simulink model "Proposed"  (R2024b)
settings: Solver=VariableStepAuto  StartTime=0.0  StopTime=1  RelTol=1e-3
undefined symbols (not defined in the file or in its folder): DiscIntNeverNeededParam, Ki, Kp, Ts
libraries: spsDiodeLib x6, spsIGBTDiodeLib x6, spsSeriesRLCBranchLib x5, powerlib_extras x3, spsThreePhaseVIMeasurementLib x3, spsSaturableTransformerLib x3, spsThreePhaseSeriesRLCBranchLib x2, spsMultimeterLib x1, spsThreePhaseProgrammableVoltageSourceLib x1, spsGroundLib x1, dspfdesign x1, spsUniversalBridgeLib x1
settings Model: VariantFading=off  Creator=skill  LastModifiedBy=skill
settings DebuggingCC: AlgebraicLoopMsg=none

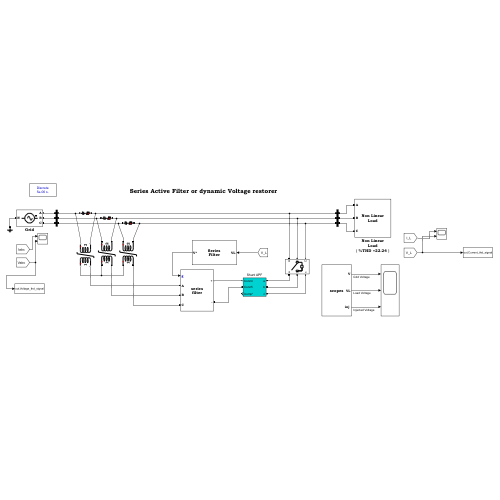
[thumbnail: Simulink's stored preview of the top-level diagram]
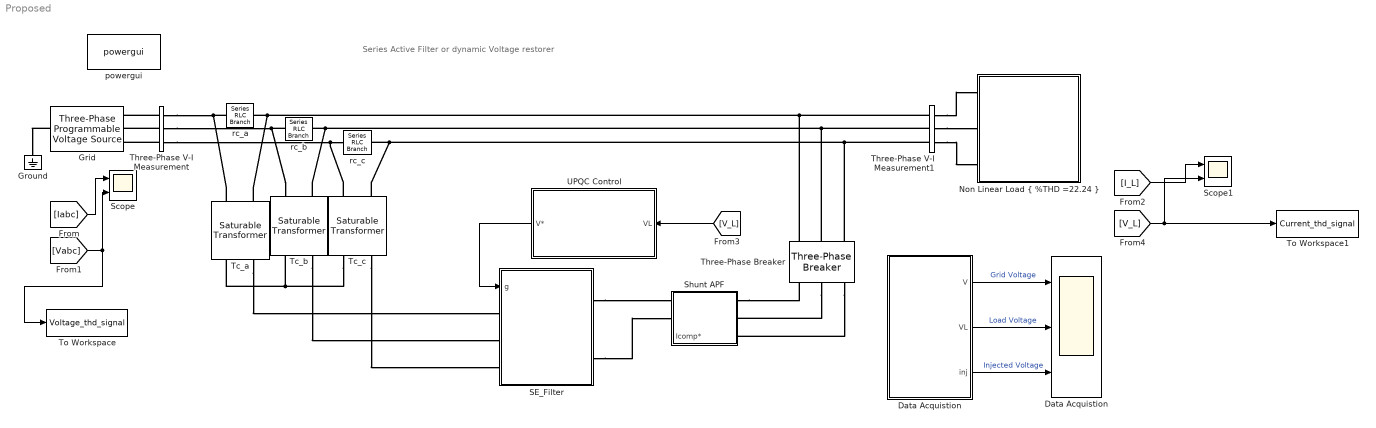
== system Proposed ==
  note: Series Active Filter or dynamic Voltage restorer
  Data Acquistion : Scope  NumInputPorts=3
  Data Acquistion : Subsystem
      mask Display: fprintf('scopes')
  Grid : spsThreePhaseProgrammableVoltageSourceLib/Three-Phase Programmable Voltage Source  PositiveSequence="[380  0 50]"  VariationEntity=Amplitude  VariationType=Table of time-amplitude pairs  VariationTypeAlt=Step  VariationStep=0.5  VariationRate=10  VariationMagnitude=0.3  VariationFrequency=2  VariationTiming=[1 2]  VariationPhaseA=off  Amplitudes=[1 0.5 1 1.5 1]  TimeValues=[0 0.5 0.7 1.5 1.7]  HarmonicGeneration=on  HarmonicA=[5 0.2 0 2]  HarmonicB=[7 0.05 0 1]  Timing="[0.2  0.4]"  BusType=swing  Pref=0  Qref=0  Qmin=-inf  Qmax=inf
  Ground : spsGroundLib/Ground  LConnTagsString=a
  "Non Linear Load { %THD =22.24 }" : Subsystem
      mask Display: fprintf('Non Linear\nLoad')
  SE_Filter : Subsystem
      mask Display: fprintf('series\nfilter')
  Scope : Scope  NumInputPorts=2
  Scope1 : Scope  NumInputPorts=2
  Shunt APF : Subsystem
      settings: PortSchema="{\"entries\":[{\"content\":{\"sides\":[{\"content\":{\"connectorIds\":[\"LConn1\",\"LConn2\",\"LConn3\"]},\"type\":\"ConnectorPlacement.EquallySpacedRectSide\",\"uuid\":\"d6bbf745-3af2-48b6-83a9-f1a4b39ae2fb\"},{\"content\":{\"connectorIds\":[\"RConn1\",\"RConn2\",\"Out1\"],\"side\":\"RIGHT\"},\"type\":\"ConnectorPlacement.EquallySpacedRectSide\",\"uuid\":\"e94a56cb-32a6-4b87-b27c-70bac7a36721\"},{\"content\":{\"side\":\"TOP\"},\"type\":\"ConnectorPlacement.EquallySpacedRectSide\",\"uuid\":\"720601aa-3b64-4420-8a99-8d6df25a17e3\"}]},\"type\":\"ConnectorPlacement.EquallySpacedConnector\",\"uuid\":\"c84ba404-e5ea-4b21-b879-47ad5a70dfc8\"}],\"packageUris\":[\"http://schema.mathworks.com/mf0/Connector/R2020b\"],\"version\":\"1.0\"}"
  Tc_a : spsSaturableTransformerLib/Saturable Transformer  ThreeWindings=off  Hysteresis=off  DataFile='hysteresis.mat'  Measurements=None  UNITS=pu  NominalPower=[4000 50]  Winding1="[380  0.02  0.02 ]"  Winding2="[380  0.02  0.02]"  Winding3="[ 315e3  0.002  0.08 ]"  Saturation=[ 0 0 ;1.016 9.043]*1e-3  CoreLoss=[117 0]  BreakLoop=off  DiscreteSolver=Trapezoidal iterative  DataType=off  InitialFlux=0  TransfoNumber=1
      settings: LibrarySourceBlock=sps_lib/Power Grid Elements/Saturable Transformer
  Tc_b : spsSaturableTransformerLib/Saturable Transformer  ThreeWindings=off  Hysteresis=off  DataFile='hysteresis.mat'  Measurements=None  UNITS=pu  NominalPower=[4000 50]  Winding1="[380  0.02  0.02 ]"  Winding2="[380  0.02  0.02]"  Winding3="[ 315e3  0.002  0.08 ]"  Saturation=[ 0 0 ;1.016 9.043]*1e-3  CoreLoss=[117 0]  BreakLoop=off  DiscreteSolver=Trapezoidal iterative  DataType=off  InitialFlux=0  TransfoNumber=1
      settings: LibrarySourceBlock=sps_lib/Power Grid Elements/Saturable Transformer
  Tc_c : spsSaturableTransformerLib/Saturable Transformer  ThreeWindings=off  Hysteresis=off  DataFile='hysteresis.mat'  Measurements=None  UNITS=pu  NominalPower=[4000 50]  Winding1="[380  0.02  0.02 ]"  Winding2="[380  0.02  0.02]"  Winding3="[ 315e3  0.002  0.08 ]"  Saturation=[ 0 0 ;1.016 9.043]*1e-3  CoreLoss=[117 0]  BreakLoop=off  DiscreteSolver=Trapezoidal iterative  DataType=off  InitialFlux=0  TransfoNumber=1
      settings: LibrarySourceBlock=sps_lib/Power Grid Elements/Saturable Transformer
  Three-Phase V-I Measurement : spsThreePhaseVIMeasurementLib/Three-Phase V-I Measurement  VoltageMeasurement=phase-to-ground  SetLabelV=on  LabelV=Vabc  Vpu=off  VpuLL=off  CurrentMeasurement=yes  SetLabelI=on  LabelI=Iabc  Ipu=off  Pbase=100e6  Vbase=500e3  OutputType=Complex  PhasorSimulation=off  PSBequivalent=0
  Three-Phase V-I Measurement1 : spsThreePhaseVIMeasurementLib/Three-Phase V-I Measurement  VoltageMeasurement=phase-to-ground  SetLabelV=on  LabelV=V_L  Vpu=off  VpuLL=off  CurrentMeasurement=yes  SetLabelI=on  LabelI=I_L  Ipu=off  Pbase=100e6  Vbase=500e3  OutputType=Complex  PhasorSimulation=off  PSBequivalent=0
  Three-Phase Breaker : spsThreePhaseBreakerLib/Three-Phase Breaker  InitialState=open  SwitchA=on  SwitchB=on  SwitchC=on  SwitchTimes=0.02  External=off  BreakerResistance=1e-6  SnubberResistance=1e6  SnubberCapacitance=inf  Measurements=None
  To Workspace : ToWorkspace  VariableName=Voltage_thd_signal  SaveFormat=Timeseries  SampleTime=-1
  To Workspace1 : ToWorkspace  VariableName=Current_thd_signal  SaveFormat=Timeseries  SampleTime=-1
  UPQC Control : Subsystem
      mask Display: fprintf('Series\nFilter')
  powergui : sps_lib/powergui  Priority=1  SimulationMode=Discrete  SampleTime=5e-6  frequency=60  Iterations=50  frequencyindice=50  Pbase=100e6  ErrMax=1e-4  UnitsV=kV  UnitsW=MW  buscounter=0  FunctionMessages=off  echomessages=off  EnableUseOfTLC=off  CurrentSourceSwitches=off  DisableSnubberDevices=off  DisableRonSwitches=off  DisableVfSwitches=off  DisplayEquations=off  AutomaticDiscreteSolvers=off  SolverType=Tustin/Backward Euler (TBE)  Interpol=off  ExternalGateDelay=off  methode=off  Ts=100  x0status=blocks  SPID=on  SwTol=0  HookPort=off  NonlinearTolerance=1e-4  nMaxIteration=100  ContinueOnMaxIteration=off  RestoreLinks=warning  ResistiveCurrentMeasurement=off  Frange=[0:2:500]  Ylog=off  Xlog=on  ShowGrid=off  save=off  variable=ZData  structure=0  ZoomFFT=off  StartTime=0.0  cycles=1  DisplayStyle=1  fundamental=60  FreqAxis=off  MaxFrequency=1000  frequencyindicesteady=1  RmsSteady=1  display=off
  rc_a : spsSeriesRLCBranchLib/Series RLC Branch  LConnTagsString=__new0  RConnTagsString=__new0  BranchType=RC  Resistance=1  Inductance=1e-3  SetiL0=off  InitialCurrent=0  Capacitance=100e-6  Setx0=off  InitialVoltage=0  Measurements=Branch voltage
  rc_b : spsSeriesRLCBranchLib/Series RLC Branch  LConnTagsString=__new0  RConnTagsString=__new0  BranchType=RC  Resistance=1  Inductance=1e-3  SetiL0=off  InitialCurrent=0  Capacitance=100e-6  Setx0=off  InitialVoltage=0  Measurements=Branch voltage
  rc_c : spsSeriesRLCBranchLib/Series RLC Branch  LConnTagsString=__new0  RConnTagsString=__new0  BranchType=RC  Resistance=1  Inductance=1e-3  SetiL0=off  InitialCurrent=0  Capacitance=100e-6  Setx0=off  InitialVoltage=0  Measurements=Branch voltage
  wires:
  Data Acquistion/1(V) -> Data Acquistion/1  "Grid Voltage"
  Data Acquistion/2(VL) -> Data Acquistion/2  "Load Voltage"
  [V_L] -> UPQC Control/1(VL)
  UPQC Control/1(V*) -> SE_Filter/1(g)
  Data Acquistion/3("inj ") -> Data Acquistion/3  "Injected Voltage"
  [Iabc] -> Scope/1
  [Vabc] -> To Workspace/1, Scope/2
  [I_L] -> Scope1/1
  [V_L] -> Scope1/2, To Workspace1/1
  connections:
  Tc_c/RConn2 -- Three-Phase Breaker/LConn3 -- Three-Phase V-I Measurement1/LConn3 -- rc_c/LConn1
  Tc_a/RConn1 -- rc_a/RConn1 -- Three-Phase V-I Measurement/RConn1
  Tc_b/LConn1 -- Tc_c/LConn1 -- Tc_a/LConn1
  Tc_c/RConn1 -- rc_c/RConn1 -- Three-Phase V-I Measurement/RConn3
  Tc_a/RConn2 -- Three-Phase Breaker/LConn1 -- Three-Phase V-I Measurement1/LConn1 -- rc_a/LConn1
  Tc_b/RConn1 -- rc_b/RConn1 -- Three-Phase V-I Measurement/RConn2
  Tc_b/RConn2 -- Three-Phase Breaker/LConn2 -- Three-Phase V-I Measurement1/LConn2 -- rc_b/LConn1
  Three-Phase V-I Measurement1/RConn3 -- "Non Linear Load { %THD =22.24 }"/LConn3
  Three-Phase V-I Measurement/LConn1 -- Grid/RConn1
  Three-Phase V-I Measurement1/RConn1 -- "Non Linear Load { %THD =22.24 }"/LConn1
  Three-Phase V-I Measurement/LConn2 -- Grid/RConn2
  Tc_c/LConn2 -- SE_Filter/LConn3
  Tc_b/LConn2 -- SE_Filter/LConn2
  Three-Phase V-I Measurement/LConn3 -- Grid/RConn3
  Tc_a/LConn2 -- SE_Filter/LConn1
  Three-Phase V-I Measurement1/RConn2 -- "Non Linear Load { %THD =22.24 }"/LConn2
  Grid/LConn1 -- Ground/LConn1
  Three-Phase Breaker/RConn2 -- Shunt APF/LConn2
  Shunt APF/LConn1 -- Three-Phase Breaker/RConn1
  Three-Phase Breaker/RConn3 -- Shunt APF/LConn3
  SE_Filter/RConn1 -- Shunt APF/RConn1
  SE_Filter/RConn2 -- Shunt APF/RConn2

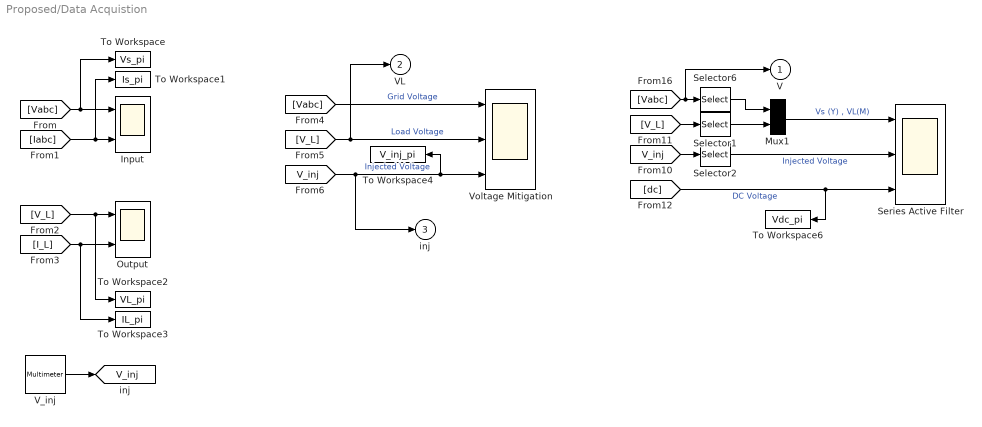
== system Proposed/Data Acquistion ==
  Input : Scope  NumInputPorts=2
  Mux1 : Mux  Inputs=2
      settings: DisplayOption=signals
  Output : Scope  NumInputPorts=2
  Selector1 : Selector  InputPortWidth=3  IndexOptions=Index vector (dialog)  Indices=1  OutputSizes=1
  Selector2 : Selector  InputPortWidth=3  IndexOptions=Index vector (dialog)  Indices=1  OutputSizes=1
  Selector6 : Selector  InputPortWidth=3  IndexOptions=Index vector (dialog)  Indices=1  OutputSizes=1
  Series Active Filter : Scope  NumInputPorts=3
  To Workspace : ToWorkspace  VariableName=Vs_pi  SampleTime=Ts
  To Workspace1 : ToWorkspace  VariableName=Is_pi  SampleTime=Ts
  To Workspace2 : ToWorkspace  VariableName=VL_pi  SampleTime=Ts
  To Workspace3 : ToWorkspace  VariableName=IL_pi  SampleTime=Ts
  To Workspace4 : ToWorkspace  VariableName=V_inj_pi  SampleTime=Ts
  To Workspace6 : ToWorkspace  VariableName=Vdc_pi  SampleTime=Ts
  V_inj : spsMultimeterLib/Multimeter  L=3  sel=[1 2 3]  yselected={}  Gain=[1 1 1]  OutputType=Complex  PlotAtSimulationStop=off  PhasorSimulation=off
  Voltage Mitigation : Scope  NumInputPorts=3
  V : Outport
  VL : Outport  Port=2
  "inj " : Outport  Port=3
  tag scope: V_inj=global
  wires:
  [Vabc] -> Input/1, To Workspace/1
  [Iabc] -> Input/2, To Workspace1/1
  [V_L] -> Output/1, To Workspace2/1
  [I_L] -> Output/2, To Workspace3/1
  [Vabc] -> Voltage Mitigation/1  "Grid Voltage"
  [V_L] -> Voltage Mitigation/2, VL/1  "Load Voltage"
  [V_inj] -> Voltage Mitigation/3, To Workspace4/1, "inj "/1  "Injected Voltage"
  [V_L] -> Selector1/1
  [V_inj] -> Selector2/1
  [dc] -> Series Active Filter/3, To Workspace6/1  "DC Voltage"
  Selector2/1 -> Series Active Filter/2  "Injected Voltage"
  [Vabc] -> Selector6/1, V/1
  Selector1/1 -> Mux1/2
  Mux1/1 -> Series Active Filter/1  "Vs (Y) , VL(M)"
  Selector6/1 -> Mux1/1
  V_inj/1 -> [V_inj]

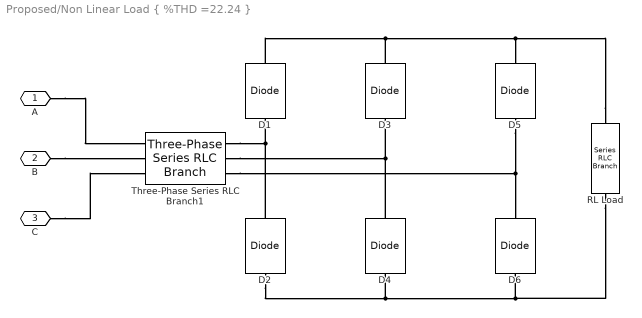
== system Proposed/Non Linear Load { %THD =22.24 } ==
  D{1..6} (6 alike) : spsDiodeLib/Diode  Ron=0.001  Lon=0  Vf=0.8  IC=0  UseSnubber=off  Rs=500  Cs=250e-9  Measurements=off
  RL Load : spsSeriesRLCBranchLib/Series RLC Branch  LConnTagsString=__new0  RConnTagsString=__new0  BranchType=RL  Resistance=60  Inductance=0.15e-3  SetiL0=off  InitialCurrent=0  Capacitance=1e-6  Setx0=off  InitialVoltage=0  Measurements=None
  Three-Phase Series RLC Branch1 : spsThreePhaseSeriesRLCBranchLib/Three-Phase Series RLC Branch  LConnTagsString=A|B|C  RConnTagsString=A|B|C  BranchType=RL  Resistance=0.4  Inductance=15e-3  Capacitance=1e-6  Measurements=None
  A : PMIOPort  Side=Left
  B : PMIOPort  Port=2  Side=Left
  C : PMIOPort  Port=3  Side=Left
  connections:
  C/RConn1 -- Three-Phase Series RLC Branch1/LConn3
  B/RConn1 -- Three-Phase Series RLC Branch1/LConn2
  A/RConn1 -- Three-Phase Series RLC Branch1/LConn1
  Three-Phase Series RLC Branch1/RConn3 -- D6/RConn1 -- D5/LConn1
  Three-Phase Series RLC Branch1/RConn2 -- D4/RConn1 -- D3/LConn1
  RL Load/RConn1 -- D6/LConn1 -- D4/LConn1 -- D2/LConn1
  RL Load/LConn1 -- D5/RConn1 -- D3/RConn1 -- D1/RConn1
  Three-Phase Series RLC Branch1/RConn1 -- D2/RConn1 -- D1/LConn1

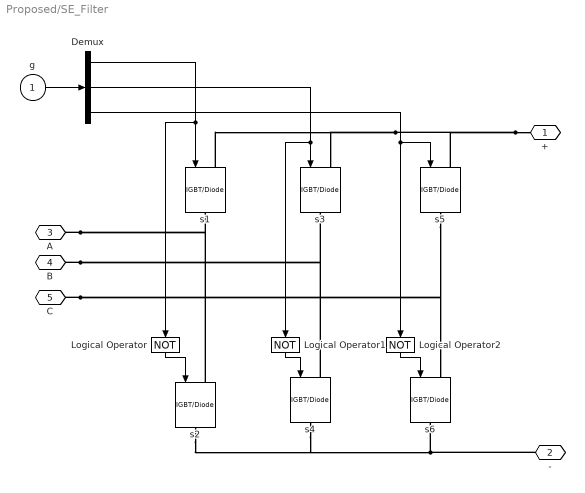
== system Proposed/SE_Filter ==
  g : Inport
  Demux : Demux  Outputs=3
      settings: DisplayOption=none
  Logical Operator : Logic  Operator=NOT  AllPortsSameDT=off  OutDataTypeStr=boolean
  Logical Operator1 : Logic  Operator=NOT  AllPortsSameDT=off  OutDataTypeStr=boolean
  Logical Operator2 : Logic  Operator=NOT  AllPortsSameDT=off  OutDataTypeStr=boolean
  s{1..6} (6 alike) : spsIGBTDiodeLib/IGBT//Diode  Ron=1e-3  Rs=1e5  Cs=inf  Measurements=off
  + : PMIOPort  Side=Right
  - : PMIOPort  Port=2  Side=Right
  A : PMIOPort  Port=3  Side=Left
  B : PMIOPort  Port=4  Side=Left
  C : PMIOPort  Port=5  Side=Left
  wires:
  Demux/2 -> s3/1, Logical Operator1/1
  Demux/1 -> s1/1, Logical Operator/1
  Logical Operator/1 -> s2/1
  Logical Operator1/1 -> s4/1
  Logical Operator2/1 -> s6/1
  Demux/3 -> Logical Operator2/1, s5/1
  g/1 -> Demux/1
  connections:
  +/RConn1 -- s5/LConn1 -- s1/LConn1 -- s3/LConn1
  A/RConn1 -- s2/LConn1 -- s1/RConn1
  -/RConn1 -- s6/RConn1 -- s4/RConn1 -- s2/RConn1
  B/RConn1 -- s4/LConn1 -- s3/RConn1
  C/RConn1 -- s5/RConn1 -- s6/LConn1

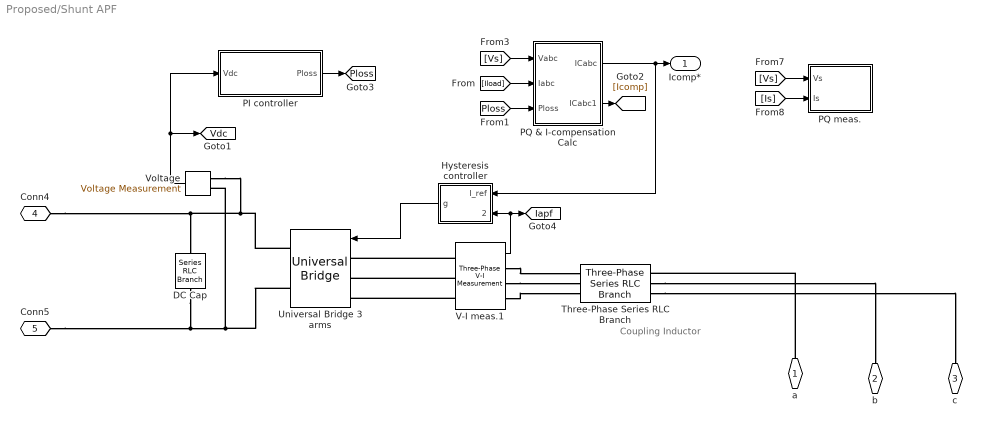
== system Proposed/Shunt APF ==
  note: Coupling Inductor
  DC Cap : spsSeriesRLCBranchLib/Series RLC Branch  LConnTagsString=__new0  RConnTagsString=__new0  BranchType=C  Resistance=1  Inductance=1e-3  SetiL0=off  InitialCurrent=0  Capacitance=3.5e-6  Setx0=off  InitialVoltage=400  Measurements=None
  Hysteresis controller : Subsystem
  PI controller : Subsystem
  PQ & I-compensation Calc : Subsystem
  PQ meas. : Subsystem
  Three-Phase Series RLC Branch : spsThreePhaseSeriesRLCBranchLib/Three-Phase Series RLC Branch  LConnTagsString=A|B|C  RConnTagsString=A|B|C  BranchType=L  Resistance=1e9  Inductance=10e-3  Capacitance=.2e-3  Measurements=None
  Universal Bridge 3 arms : spsUniversalBridgeLib/Universal Bridge  Arms=3  SnubberResistance=10000  SnubberCapacitance=inf  Device=IGBT / Diodes  Ron=1e-4  Lon=0  ForwardVoltages="[  1  1  ]"  ForwardVoltage=.8  GTOparameters=[ 10e-6 , 20e-6 ]  IGBTparameters=[ 1e-6 , 2e-6 ]  Measurements=None  Measurements_2=None  converterType=Rectifier
      settings: AttributesFormatString=\n
  V-I meas.1 : spsThreePhaseVIMeasurementLib/Three-Phase V-I Measurement  VoltageMeasurement=phase-to-ground  SetLabelV=on  LabelV=Vnm  Vpu=off  VpuLL=off  CurrentMeasurement=yes  SetLabelI=off  LabelI=Iabc  Ipu=off  Pbase=100e6  Vbase=500e3  OutputType=Complex  PhasorSimulation=off  PSBequivalent=0
  Voltage : spsVoltageMeasurementLib/Voltage Measurement  PhasorSimulation=off  OutputType=Complex  PSBequivalent=0
  a : PMIOPort  Side=Left
  b : PMIOPort  Port=2  Side=Left
  c : PMIOPort  Port=3  Side=Left
  Conn4 : PMIOPort  Port=4  Side=Right
  Conn5 : PMIOPort  Port=5  Side=Right
  Icomp* : Outport
  tag scope: Iapf=global, Ploss=global, Vdc=global
  wires:
  [Iload] -> PQ & I-compensation Calc/2(Iabc)
  V-I meas.1/1 -> Hysteresis controller/2(I_meas), [Iapf]
  Hysteresis controller/1(g) -> Universal Bridge 3 arms/1
  PQ & I-compensation Calc/1(ICabc) -> Hysteresis controller/1(I_ref), Icomp*/1
  Voltage/1 -> PI controller/1(Vdc), [Vdc]
  [Vs] -> PQ & I-compensation Calc/1(Vabc)
  PQ & I-compensation Calc/2(ICabc1) -> [Icomp]
  PI controller/1(Ploss) -> [Ploss]
  [Ploss] -> PQ & I-compensation Calc/3(Ploss)
  [Vs] -> PQ meas./1(Vs)
  [Is] -> PQ meas./2(Is)
  connections:
  Voltage/LConn1 -- DC Cap/LConn1 -- Conn4/RConn1 -- Universal Bridge 3 arms/RConn1
  V-I meas.1/LConn1 -- Universal Bridge 3 arms/LConn1
  V-I meas.1/LConn2 -- Universal Bridge 3 arms/LConn2
  V-I meas.1/RConn3 -- Three-Phase Series RLC Branch/LConn3
  V-I meas.1/RConn2 -- Three-Phase Series RLC Branch/LConn2
  V-I meas.1/LConn3 -- Universal Bridge 3 arms/LConn3
  V-I meas.1/RConn1 -- Three-Phase Series RLC Branch/LConn1
  a/RConn1 -- Three-Phase Series RLC Branch/RConn1
  Three-Phase Series RLC Branch/RConn2 -- b/RConn1
  Three-Phase Series RLC Branch/RConn3 -- c/RConn1
  DC Cap/RConn1 -- Conn5/RConn1 -- Universal Bridge 3 arms/RConn2 -- Voltage/LConn2

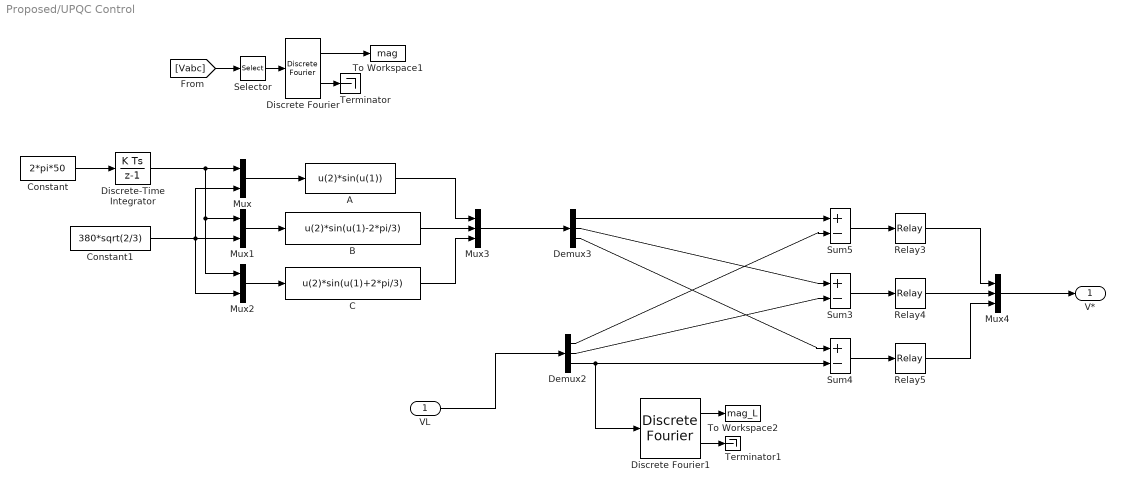
== system Proposed/UPQC Control ==
  VL : Inport
  A : Fcn  Expr=u(2)*sin(u(1))
  B : Fcn  Expr=u(2)*sin(u(1)-2*pi/3)
  C : Fcn  Expr=u(2)*sin(u(1)+2*pi/3)
  Constant : Constant  Value=2*pi*50
  Constant1 : Constant  Value=380*sqrt(2/3)
  Demux2 : Demux  Outputs=3
  Demux3 : Demux  Outputs=3
  Discrete Fourier : powerlib_extras/Discrete Measurements/Discrete  Fourier  Freq=50  n=1  Par_Init=[0 0]  Ts=Ts
  Discrete Fourier1 : powerlib_extras/Discrete Measurements/Discrete  Fourier  Freq=50  n=1  Par_Init=[0 0]  Ts=Ts
  Discrete-Time Integrator : DiscreteIntegrator  gainval=Gain  SampleTime=Ts  ICPrevOutput=DiscIntNeverNeededParam  ICPrevScaledInput=DiscIntNeverNeededParam
  Mux : Mux  Inputs=2
  Mux1 : Mux  Inputs=2
  Mux2 : Mux  Inputs=2
  Mux3 : Mux  Inputs=3
  Mux4 : Mux  Inputs=3
  Relay3 : Relay  OnSwitchValue=1  OffSwitchValue=-1
  Relay4 : Relay  OnSwitchValue=1  OffSwitchValue=-1
  Relay5 : Relay  OnSwitchValue=1  OffSwitchValue=-1
  Selector : Selector  InputPortWidth=3  IndexOptions=Index vector (dialog)  Indices=1  OutputSizes=1
  Sum3 : Sum  Inputs=+-
  Sum4 : Sum  Inputs=+-
  Sum5 : Sum  Inputs=+-
  Terminator : Terminator
  Terminator1 : Terminator
  To Workspace1 : ToWorkspace  VariableName=mag  SampleTime=Ts
  To Workspace2 : ToWorkspace  VariableName=mag_L  SampleTime=Ts
  V* : Outport
  wires:
  Constant/1 -> Discrete-Time Integrator/1
  Discrete-Time Integrator/1 -> Mux/1, Mux2/1, Mux1/1
  Constant1/1 -> Mux1/2, Mux2/2, Mux/2
  Mux/1 -> A/1
  Mux1/1 -> B/1
  Mux2/1 -> C/1
  Discrete Fourier/2 -> Terminator/1
  Selector/1 -> Discrete Fourier/1
  [Vabc] -> Selector/1
  Discrete Fourier/1 -> To Workspace1/1
  A/1 -> Mux3/1
  B/1 -> Mux3/2
  C/1 -> Mux3/3
  Discrete Fourier1/2 -> Terminator1/1
  Sum5/1 -> Relay3/1
  Sum3/1 -> Relay4/1
  Sum4/1 -> Relay5/1
  Relay3/1 -> Mux4/1
  Relay4/1 -> Mux4/2
  Relay5/1 -> Mux4/3
  Mux4/1 -> V*/1
  Discrete Fourier1/1 -> To Workspace2/1
  VL/1 -> Demux2/1
  Demux3/1 -> Sum5/1
  Demux2/3 -> Sum4/2, Discrete Fourier1/1
  Demux2/1 -> Sum5/2
  Demux3/3 -> Sum4/1
  Demux2/2 -> Sum3/2
  Demux3/2 -> Sum3/1
  Mux3/1 -> Demux3/1

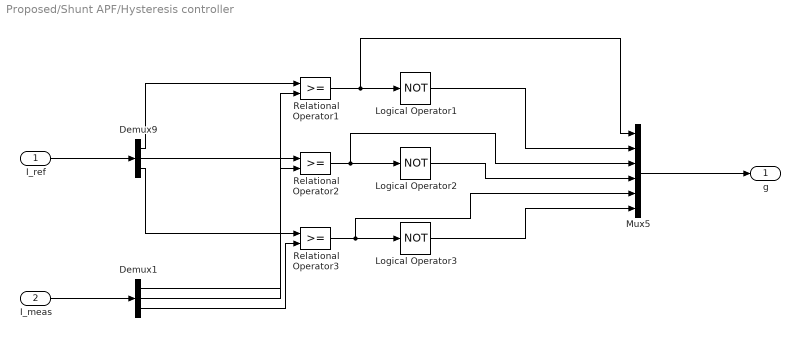
== system Proposed/Shunt APF/Hysteresis controller ==
  I_ref : Inport
  I_meas : Inport  Port=2
  Demux1 : Demux  Outputs=3
  Demux9 : Demux  Outputs=3
  Logical Operator1 : Logic  Operator=NOT  AllPortsSameDT=off  OutDataTypeStr=boolean
  Logical Operator2 : Logic  Operator=NOT  AllPortsSameDT=off  OutDataTypeStr=boolean
  Logical Operator3 : Logic  Operator=NOT  AllPortsSameDT=off  OutDataTypeStr=boolean
  Mux5 : Mux  Inputs=6
  Relational Operator1 : RelationalOperator  OutDataTypeStr=boolean  InputSameDT=off
  Relational Operator2 : RelationalOperator  OutDataTypeStr=boolean  InputSameDT=off
  Relational Operator3 : RelationalOperator  OutDataTypeStr=boolean  InputSameDT=off
  g : Outport
  wires:
  Relational Operator1/1 -> Logical Operator1/1, Mux5/1
  Relational Operator2/1 -> Logical Operator2/1, Mux5/3
  Relational Operator3/1 -> Logical Operator3/1, Mux5/5
  Demux9/1 -> Relational Operator1/1
  Demux9/3 -> Relational Operator3/1
  Logical Operator1/1 -> Mux5/2
  Logical Operator2/1 -> Mux5/4
  Logical Operator3/1 -> Mux5/6
  Mux5/1 -> g/1
  Demux9/2 -> Relational Operator2/1
  Demux1/1 -> Relational Operator1/2
  Demux1/2 -> Relational Operator2/2
  Demux1/3 -> Relational Operator3/2
  I_ref/1 -> Demux9/1
  I_meas/1 -> Demux1/1

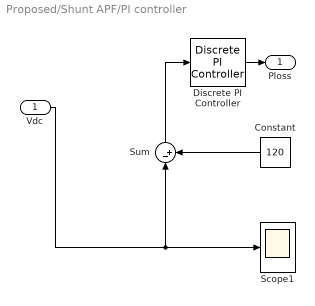
== system Proposed/Shunt APF/PI controller ==
  Vdc : Inport
  Constant : Constant  Value=120
  Discrete PI Controller : powerlib_extras/Discrete  Control Blocks/Discrete PI Controller  Kp=Kp  Ki=Ki  Par_Limits=[1e6 -1e6]  Init=0  Ts=5e-6
  Scope1 : Scope
  Sum : Sum  Inputs=|-+
  Ploss : Outport
  wires:
  Constant/1 -> Sum/2
  Sum/1 -> Discrete PI Controller/1
  Discrete PI Controller/1 -> Ploss/1
  Vdc/1 -> Sum/1, Scope1/1

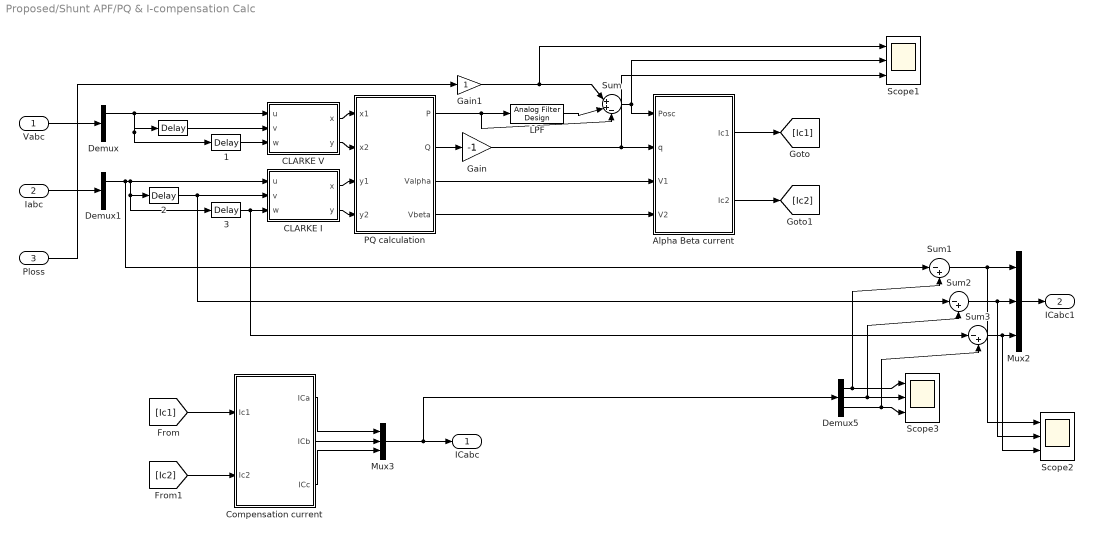
== system Proposed/Shunt APF/PQ & I-compensation Calc ==
  Vabc : Inport
  Iabc : Inport  Port=2
  Ploss : Inport  Port=3
  " " : TransportDelay  DelayTime=0.006666666  BufferSize=6890
  " 1" : TransportDelay  DelayTime=0.013333333  BufferSize=77889
  " 2" : TransportDelay  DelayTime=0.006666666  BufferSize=6789
  " 3" : TransportDelay  DelayTime=0.013333333  BufferSize=5667
  Alpha Beta current : MATLAB Function  TreatAsAtomicUnit=on
  CLARKE I : MATLAB Function  TreatAsAtomicUnit=on
  CLARKE V : MATLAB Function  TreatAsAtomicUnit=on
  Compensation current : MATLAB Function  TreatAsAtomicUnit=on
  Demux : Demux  Outputs=3
  Demux1 : Demux  Outputs=3
  Demux5 : Demux  Outputs=3
  Gain : Gain  Gain=-1
  Gain1 : Gain
  LPF : dspfdesign/Analog Filter Design  method=Butterworth  filttype=Lowpass  N=5  Wlo=2*pi*50  Whi=80  Rp=2  Rs=40
  Mux2 : Mux  Inputs=3
  Mux3 : Mux  Inputs=3
  PQ calculation : MATLAB Function  TreatAsAtomicUnit=on
  Scope1 : Scope  NumInputPorts=3
  Scope2 : Scope  NumInputPorts=3
  Scope3 : Scope  NumInputPorts=3
  Sum : Sum  Inputs=|++-
  Sum1 : Sum  Inputs=|-+
  Sum2 : Sum  Inputs=|-+
  Sum3 : Sum  Inputs=|-+
  ICabc : Outport
  ICabc1 : Outport  Port=2
  wires:
  Iabc/1 -> Demux1/1
  Vabc/1 -> Demux/1
  [Ic1] -> Compensation current/1(Ic1)
  [Ic2] -> Compensation current/2(Ic2)
  Compensation current/1(ICa) -> Mux3/1
  Compensation current/2(ICb) -> Mux3/2
  Compensation current/3(ICc) -> Mux3/3
  CLARKE V/1(x) -> PQ calculation/1(x1)
  CLARKE V/2(y) -> PQ calculation/2(x2)
  CLARKE I/1(x) -> PQ calculation/3(y1)
  PQ calculation/2(Q) -> Gain/1
  PQ calculation/1(P) -> LPF/1, Sum/3
  Gain/1 -> Alpha Beta current/2(q), Scope1/3
  PQ calculation/3(Valpha) -> Alpha Beta current/3(V1)
  Alpha Beta current/1(Ic1) -> [Ic1]
  Alpha Beta current/2(Ic2) -> [Ic2]
  CLARKE I/2(y) -> PQ calculation/4(y2)
  PQ calculation/4(Vbeta) -> Alpha Beta current/4(V2)
  Demux/1 -> CLARKE V/1(u), " "/1, " 1"/1
  Demux1/1 -> Sum1/1, CLARKE I/1(u), " 3"/1, " 2"/1
  LPF/1 -> Sum/2
  Sum/1 -> Alpha Beta current/1(Posc), Scope1/2
  Gain1/1 -> Sum/1, Scope1/1
  Mux3/1 -> ICabc/1, Demux5/1
  Demux5/1 -> Scope3/1, Sum1/2
  Demux5/2 -> Scope3/2, Sum2/2
  Demux5/3 -> Scope3/3, Sum3/2
  Ploss/1 -> Gain1/1
  Sum1/1 -> Mux2/1, Scope2/1
  Sum2/1 -> Mux2/2, Scope2/2
  Sum3/1 -> Mux2/3, Scope2/3
  Mux2/1 -> ICabc1/1
  " "/1 -> CLARKE V/2(v)
  " 1"/1 -> CLARKE V/3(w)
  " 2"/1 -> CLARKE I/2(v), Sum2/1
  " 3"/1 -> CLARKE I/3(w), Sum3/1

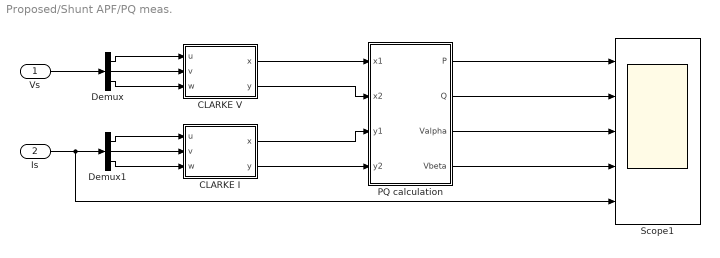
== system Proposed/Shunt APF/PQ meas. ==
  Vs : Inport
  Is : Inport  Port=2
  CLARKE I : MATLAB Function  TreatAsAtomicUnit=on
  CLARKE V : MATLAB Function  TreatAsAtomicUnit=on
  Demux : Demux  Outputs=3
  Demux1 : Demux  Outputs=3
  PQ calculation : MATLAB Function  TreatAsAtomicUnit=on
  Scope1 : Scope  NumInputPorts=5
  wires:
  CLARKE V/1(x) -> PQ calculation/1(x1)
  CLARKE V/2(y) -> PQ calculation/2(x2)
  CLARKE I/1(x) -> PQ calculation/3(y1)
  CLARKE I/2(y) -> PQ calculation/4(y2)
  Demux/1 -> CLARKE V/1(u)
  Demux/2 -> CLARKE V/2(v)
  Demux/3 -> CLARKE V/3(w)
  Demux1/1 -> CLARKE I/1(u)
  Demux1/2 -> CLARKE I/2(v)
  Demux1/3 -> CLARKE I/3(w)
  Vs/1 -> Demux/1
  Is/1 -> Demux1/1, Scope1/5
  PQ calculation/1(P) -> Scope1/1
  PQ calculation/2(Q) -> Scope1/2
  PQ calculation/3(Valpha) -> Scope1/3
  PQ calculation/4(Vbeta) -> Scope1/4

== matlab function Proposed/Shunt APF/PQ & I-compensation Calc/CLARKE I ==
  data: u input; x output; v input; w input; y output
function [x,y] = ICT(u,v,w)
%#em1

x = sqrt(2/3)*(u-(0.5*v)-(0.5*w));
y = sqrt(2)*(0+(0.5*v)-(0.5*w));

== matlab function Proposed/Shunt APF/PQ & I-compensation Calc/CLARKE V ==
  data: u input; x output; v input; w input; y output
function [x,y] = VCT(u,v,w)
%#em1

x = sqrt(2/3)*(u-(0.5*v)-(0.5*w));
y = sqrt(2)*(0+(0.5*v)-(0.5*w));

== matlab function Proposed/Shunt APF/PQ & I-compensation Calc/PQ calculation ==
  data: x1 input; P output; Q output; x2 input; y1 input; y2 input; Valpha output; Vbeta output
function [P,Q,Valpha,Vbeta] = PQ(x1,x2,y1,y2)
%#em1

P = (x1*y1)+(x2*y2);
Q = (x2*y1)-(x1*y2);
Valpha = x1;
Vbeta = x2;

== matlab function Proposed/Shunt APF/PQ & I-compensation Calc/Compensation current ==
  data: Ic1 input; ICa output; Ic2 input; ICb output; ICc output
function [ICa,ICb,ICc] = Ical(Ic1,Ic2)
%#em1

ICa = sqrt(2/3)*(Ic1);
ICb = sqrt(2/3)*((-0.5*Ic1)+((sqrt(3)/2)*Ic2));
ICc = sqrt(2/3)*((-0.5*Ic1)-((sqrt(3)/2)*Ic2));

== matlab function Proposed/Shunt APF/PQ & I-compensation Calc/Alpha Beta current ==
  data: Posc input; Ic1 output; q input; V1 input; Ic2 output; V2 input
function [Ic1,Ic2] = ICOM(Posc,q,V1,V2)
%#em1

Ic1 = (-1/(V1^2 + V2^2))*((Posc*V1)+(q*V2));
Ic2 = (-1/(V1^2 + V2^2))*((Posc*V2)-(q*V1));

== matlab function Proposed/Shunt APF/PQ meas./CLARKE I ==
  data: u input; x output; v input; w input; y output
function [x,y] = ICT(u,v,w)
%#em1

x = sqrt(2/3)*(u-(0.5*v)-(0.5*w));
y = sqrt(2)*(0+(0.5*v)-(0.5*w));

== matlab function Proposed/Shunt APF/PQ meas./CLARKE V ==
  data: u input; x output; v input; w input; y output
function [x,y] = VCT(u,v,w)
%#em1

x = sqrt(2/3)*(u-(0.5*v)-(0.5*w));
y = sqrt(2)*(0+(0.5*v)-(0.5*w));

== matlab function Proposed/Shunt APF/PQ meas./PQ calculation ==
  data: x1 input; P output; Q output; x2 input; y1 input; y2 input; Valpha output; Vbeta output
function [P,Q,Valpha,Vbeta] = PQ(x1,x2,y1,y2)
%#em1

P = (x1*y1)+(x2*y2);
Q = (x2*y1)-(x1*y2);
Valpha = x1;
Vbeta = x2;
